simulink model "DAB_variableload"  (R2024b)
settings: Solver=VariableStepAuto  StartTime=0.0  StopTime=1  RelTol=1e-3
undefined symbols (not defined in the file): sigbuilder_block
libraries: spsMosfetLib x16, spsVoltageMeasurementLib x9, spsSeriesRLCBranchLib x7, spsCurrentMeasurementLib x6, simulink x5, slpidlib x4, spsMeanLib x4, spsParallelRLCBranchLib x4, spsRMSLib x4, spsDCVoltageSourceLib x2, spsLinearTransformerLib x2, spsControlledCurrentSourceLib x1
settings Model: Creator=shiekhsoliha  LastModifiedBy=sheikhsoliha
settings SolverCC: AlgebraicLoopSolver=TrustRegion
settings DataIOCC: ReturnWorkspaceOutputs=off
settings OptimizationCC: ReuseModelBlockBuffer=off  EfficientMapNaN2IntZero=off  AccelVerboseBuild=on
settings DebuggingCC: UnconnectedInputMsg=warning  UnconnectedOutputMsg=warning  UnconnectedLineMsg=warning  ArithmeticOperatorsInVariantConditions=warning
settings HardwareCC: TargetBitPerLong=64  TargetBitPerPointer=64  TargetBitPerSizeT=64  TargetBitPerPtrDiffT=64  TargetLongLongMode=on  TargetIntDivRoundTo=Zero  TargetEndianess=LittleEndian  TargetWordSize=64  TargetHWDeviceType=MATLAB Host  ProdEqTarget=off
settings ModelReferenceCC: EnableRefExpFcnMdlSchedulingChecks=on
settings SFSimCC: SimUseLocalCustomCode=off  CustomCodeUndefinedFunction=UseInterfaceOnly
settings RTWCC: RTWUseLocalCustomCode=off  GPUComputeCapability=3.5
settings CodeAppCC: MaxIdLength=128
settings GRTTargetCC: TargetLangStandard=C89/C90 (ANSI)  CombineOutputUpdateFcns=off  GRTInterface=on

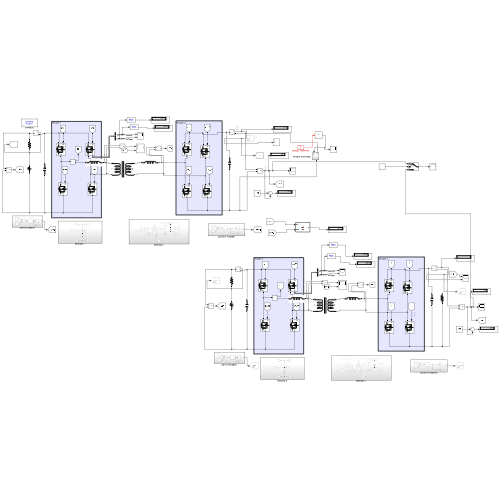
[thumbnail: Simulink's stored preview of the top-level diagram]
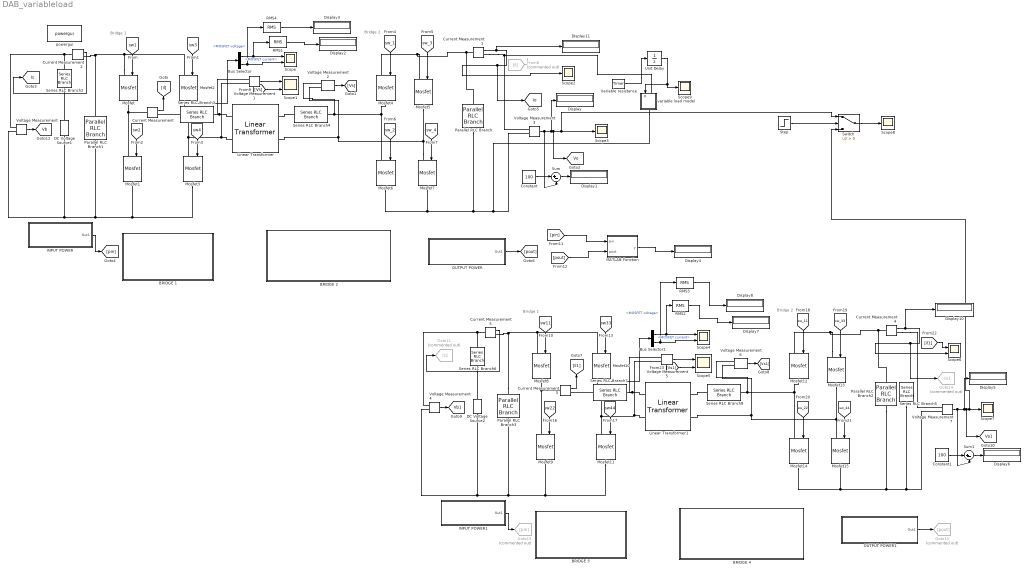
== system DAB_variableload ==
  note: Bridge 1
  note: Bridge 2
  note: Bridge 2
  note: Bridge 1
  " variable load model" : Subsystem
  BRIDGE 1 : Subsystem
  BRIDGE 2 : Subsystem
  BRIDGE 3 : Subsystem
  BRIDGE 4 : Subsystem
  Bus Selector : BusSelector  OutputSignals=MOSFET current,MOSFET voltage
  Bus Selector1 : BusSelector  OutputSignals=MOSFET current,MOSFET voltage
  Constant : Constant  Value=100
  Constant1 : Constant  Value=100
  Current Measurement{,1..5} (6 alike) : spsCurrentMeasurementLib/Current Measurement  PhasorSimulation=off  OutputType=Complex  PSBequivalent=0
  DC Voltage Source1 : spsDCVoltageSourceLib/DC Voltage Source  Amplitude=800  Measurements=None
  DC Voltage Source2 : spsDCVoltageSourceLib/DC Voltage Source  Amplitude=800  Measurements=None
  Display{,1..8,10..11} (11 alike) : Display
  From8 : From  Commented=on  GotoTag=il
  Goto11 : Goto  Commented=on  GotoTag=Is1  TagVisibility=global
  Goto13 : Goto  Commented=on  GotoTag=pin
  Goto14 : Goto  Commented=on  GotoTag=Io1  TagVisibility=global
  Goto15 : Goto  Commented=on  GotoTag=pout
  INPUT POWER : Subsystem
  INPUT POWER1 : Subsystem
  Linear Transformer : spsLinearTransformerLib/Linear Transformer  UNITS=pu  NominalPower=[ 2.5e3 50e3 ]  winding1=[1 0 0]  winding2=[1 0 0 ]  ThreeWindings=off  winding3=[ 315e3 0.002 0.08 ]  RmLm=[ 1e6 1e6 ]  Measurements=None  DataType=off
  Linear Transformer1 : spsLinearTransformerLib/Linear Transformer  UNITS=pu  NominalPower=[ 2.5e3 50e3 ]  winding1=[1 0 0]  winding2=[1 0 0 ]  ThreeWindings=off  winding3=[ 315e3 0.002 0.08 ]  RmLm=[ 1e6 1e6 ]  Measurements=None  DataType=off
  MATLAB Function : MATLAB Function  TreatAsAtomicUnit=on
  Mosfet{,1,3..9,11..15} (14 alike) : spsMosfetLib/Mosfet  Ron=0.1  Lon=0  Rd=0.01  Vfd=0  IC=0  Rs=1e5  Cs=inf  Measurements=off
  Mosfet10 : spsMosfetLib/Mosfet  Ron=0.1  Lon=0  Rd=0.01  Vfd=0  IC=0  Rs=1e5  Cs=inf  Measurements=on
  Mosfet2 : spsMosfetLib/Mosfet  Ron=0.1  Lon=0  Rd=0.01  Vfd=0  IC=0  Rs=1e5  Cs=inf  Measurements=on
  OUTPUT POWER : Subsystem
  OUTPUT POWER1 : Subsystem
  Parallel RLC Branch{,1..3} (4 alike) : spsParallelRLCBranchLib/Parallel RLC Branch  LConnTagsString=a  RConnTagsString=__new0  BranchType=C  Resistance=72.2  Inductance=1e-3  SetiL0=off  InitialCurrent=0  Capacitance=1.8e-3  Setx0=off  InitialVoltage=0  Measurements=None
  RMS{1..4} (4 alike) : spsRMSLib/RMS  TrueRMS=on  Freq=60  RMSInit=120  Ts=0
  Scope{,1,4..6} (5 alike) : Scope  NumInputPorts=2
  Scope{2..3,7..9} (5 alike) : Scope
  Series RLC Branch2 : spsSeriesRLCBranchLib/Series RLC Branch  LConnTagsString=__new0  RConnTagsString=__new0  BranchType=R  Resistance=0.1  Inductance=1e-3  SetiL0=off  InitialCurrent=0  Capacitance=1e-6  Setx0=off  InitialVoltage=0  Measurements=None
  Series RLC Branch{3..4,7..8} (4 alike) : spsSeriesRLCBranchLib/Series RLC Branch  LConnTagsString=__new0  RConnTagsString=__new0  BranchType=L  Resistance=0.1  Inductance=9.8e-6  SetiL0=off  InitialCurrent=0  Capacitance=1e-6  Setx0=off  InitialVoltage=0  Measurements=None
  Series RLC Branch5 : spsSeriesRLCBranchLib/Series RLC Branch  LConnTagsString=__new0  RConnTagsString=__new0  BranchType=R  Resistance=15  Inductance=1e-3  SetiL0=off  InitialCurrent=0  Capacitance=1e-6  Setx0=off  InitialVoltage=0  Measurements=None
  Series RLC Branch6 : spsSeriesRLCBranchLib/Series RLC Branch  LConnTagsString=__new0  RConnTagsString=__new0  BranchType=R  Resistance=0.1  Inductance=1e-3  SetiL0=off  InitialCurrent=0  Capacitance=1e-6  Setx0=off  InitialVoltage=0  Measurements=None
  Step : Step  Time=0.17  SampleTime=0
  Sum : Sum  Inputs=|+-
  Sum1 : Sum  Inputs=|+-
  Switch : Switch  Criteria=u2 > Threshold  SaturateOnIntegerOverflow=off  InputSameDT=off
  Unit Delay : UnitDelay  SampleTime=-1  HasFrameUpgradeWarning=on
  Variable resistance : powerlib_extras/Control  Blocks/Timer  t="[0  0.5 1]"  e=[31.2 15 15]
  Voltage Measurement{,1..7} (8 alike) : spsVoltageMeasurementLib/Voltage Measurement  PhasorSimulation=off  OutputType=Complex  PSBequivalent=0
  powergui : sps_lib/powergui  Priority=1  SimulationMode=Discrete  SampleTime=10e-7  frequency=60  Iterations=50  frequencyindice=0  Pbase=100e6  ErrMax=1e-4  UnitsV=kV  UnitsW=MW  buscounter=0  FunctionMessages=off  echomessages=off  EnableUseOfTLC=off  CurrentSourceSwitches=off  DisableSnubberDevices=off  DisableRonSwitches=off  DisableVfSwitches=off  DisplayEquations=off  AutomaticDiscreteSolvers=off  SolverType=Tustin/Backward Euler (TBE)  Interpol=off  ExternalGateDelay=off  methode=off  Ts=100  x0status=blocks  SPID=on  SwTol=0  HookPort=off  NonlinearTolerance=1e-4  nMaxIteration=100  ContinueOnMaxIteration=off  RestoreLinks=warning  ResistiveCurrentMeasurement=off  Frange=[0:2:500]  Ylog=off  Xlog=on  ShowGrid=off  save=off  variable=ZData  structure=0  ZoomFFT=off  StartTime=0.0  cycles=1  DisplayStyle=1  fundamental=60  FreqAxis=off  MaxFrequency=1000  frequencyindicesteady=1  RmsSteady=1  display=off
  tag scope: Io=global, Is=global, Vb1=global, Vb=global, Vo1=global, Vo=global
  wires:
  Voltage Measurement1/1 -> Scope1/1
  [sw_1] -> Mosfet4/1
  [sw_4] -> Mosfet7/1
  [sw_2] -> Mosfet6/1
  From8/1 -> ?
  [sw3] -> Mosfet2/1
  [sw_3] -> Mosfet5/1
  [Vs] -> Scope1/2
  Current Measurement/1 -> [il]
  [sw4] -> Mosfet3/1
  [sw1] -> Mosfet/1
  [sw2] -> Mosfet1/1
  Voltage Measurement2/1 -> [Vs]
  Voltage Measurement/1 -> [Vb]
  Constant/1 -> Sum/1
  Sum/1 -> Display1/1
  Mosfet2/1 -> Bus Selector/1
  Bus Selector/1 -> RMS1/1, Scope/1  "<MOSFET current>"
  Bus Selector/2 -> RMS4/1, Scope/2  "<MOSFET voltage>"
  RMS1/1 -> Display2/1
  RMS4/1 -> Display3/1
  Current Measurement2/1 -> [Is]
  INPUT POWER/1(Out1) -> [pin]
  OUTPUT POWER/1(Out1) -> [pout]
  [pin] -> MATLAB Function/1(pin)
  [pout] -> MATLAB Function/2(pout)
  MATLAB Function/1(y) -> Display4/1
  Voltage Measurement3/1 -> Sum/2, Display/1, [Vo], Switch/1, Scope3/1
  Step/1 -> Switch/2
  Voltage Measurement7/1 -> Sum1/2, Display5/1, [Vo1], Switch/3, Scope7/1
  [sw_11] -> Mosfet12/1
  [sw_22] -> Mosfet14/1
  Constant1/1 -> Sum1/1
  [sw11] -> Mosfet8/1
  [Vs1] -> Scope5/2
  Current Measurement3/1 -> [il1]
  Voltage Measurement5/1 -> Scope5/1
  Voltage Measurement4/1 -> [Vb1]
  [sw22] -> Mosfet9/1
  INPUT POWER1/1(Out1) -> Goto13/1
  Voltage Measurement6/1 -> [Vs1]
  Current Measurement5/1 -> Goto11/1
  OUTPUT POWER1/1(Out1) -> Goto15/1
  [il1] -> Scope6/1
  Current Measurement4/1 -> Display10/1, Goto14/1, Scope6/2
  [sw44] -> Mosfet11/1
  [sw_33] -> Mosfet13/1
  [sw_44] -> Mosfet15/1
  Mosfet10/1 -> Bus Selector1/1
  RMS2/1 -> Display7/1
  [sw33] -> Mosfet10/1
  Bus Selector1/2 -> RMS3/1, Scope4/2  "<MOSFET voltage>"
  RMS3/1 -> Display8/1
  Sum1/1 -> Display6/1
  Bus Selector1/1 -> RMS2/1, Scope4/1  "<MOSFET current>"
  Switch/1 -> Scope8/1
  Variable resistance/1 -> Unit Delay/1
  Unit Delay/1 -> Scope9/1, " variable load model"/1(R)
  Current Measurement1/1 -> Display11/1, [Io], Scope2/1
  connections:
  Mosfet/RConn1 -- Mosfet1/LConn1 -- Current Measurement/LConn1
  Mosfet2/RConn1 -- Voltage Measurement1/LConn2 -- Linear Transformer/LConn2 -- Mosfet3/LConn1
  Mosfet/LConn1 -- Mosfet2/LConn1 -- Current Measurement2/RConn1 -- Parallel RLC Branch1/LConn1
  Parallel RLC Branch1/RConn1 -- Voltage Measurement/LConn2 -- DC Voltage Source1/LConn1 -- Mosfet1/RConn1 -- Mosfet3/RConn1
  Current Measurement1/RConn1 -- " variable load model"/LConn1 -- Voltage Measurement3/LConn1
  Mosfet7/RConn1 -- Mosfet6/RConn1 -- Parallel RLC Branch/RConn1 -- " variable load model"/RConn1 -- Voltage Measurement3/LConn2
  Mosfet7/LConn1 -- Mosfet5/RConn1 -- Voltage Measurement2/LConn2 -- Linear Transformer/RConn2
  Voltage Measurement1/LConn1 -- Linear Transformer/LConn1 -- Series RLC Branch3/RConn1
  Series RLC Branch2/RConn1 -- DC Voltage Source1/RConn1
  Mosfet4/LConn1 -- Parallel RLC Branch/LConn1 -- Current Measurement1/LConn1 -- Mosfet5/LConn1
  Series RLC Branch3/LConn1 -- Current Measurement/RConn1
  Voltage Measurement2/LConn1 -- Mosfet6/LConn1 -- Mosfet4/RConn1 -- Series RLC Branch4/RConn1
  Series RLC Branch4/LConn1 -- Linear Transformer/RConn1
  Voltage Measurement/LConn1 -- Series RLC Branch2/LConn1 -- Current Measurement2/LConn1
  Mosfet11/LConn1 -- Mosfet10/RConn1 -- Voltage Measurement5/LConn2 -- Linear Transformer1/LConn2
  Mosfet13/LConn1 -- Mosfet12/LConn1 -- Parallel RLC Branch2/LConn1 -- Current Measurement4/LConn1
  Voltage Measurement6/LConn1 -- Series RLC Branch8/RConn1 -- Mosfet14/LConn1 -- Mosfet12/RConn1
  Voltage Measurement7/LConn2 -- Mosfet15/RConn1 -- Mosfet14/RConn1 -- Parallel RLC Branch2/RConn1 -- Series RLC Branch5/RConn1
  Linear Transformer1/RConn2 -- Mosfet15/LConn1 -- Mosfet13/RConn1 -- Voltage Measurement6/LConn2
  Current Measurement5/LConn1 -- Voltage Measurement4/LConn1 -- Series RLC Branch6/LConn1
  Current Measurement4/RConn1 -- Voltage Measurement7/LConn1
  DC Voltage Source2/LConn1 -- Parallel RLC Branch3/RConn1 -- Mosfet9/RConn1 -- Mosfet11/RConn1 -- Voltage Measurement4/LConn2
  Parallel RLC Branch3/LConn1 -- Current Measurement5/RConn1 -- Mosfet8/LConn1 -- Mosfet10/LConn1
  Series RLC Branch7/RConn1 -- Voltage Measurement5/LConn1 -- Linear Transformer1/LConn1
  Current Measurement3/LConn1 -- Mosfet8/RConn1 -- Mosfet9/LConn1
  Series RLC Branch6/RConn1 -- DC Voltage Source2/RConn1
  Series RLC Branch7/LConn1 -- Current Measurement3/RConn1
  Series RLC Branch8/LConn1 -- Linear Transformer1/RConn1

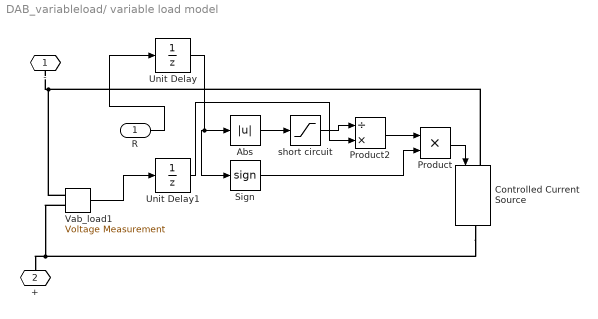
== system DAB_variableload/ variable load model ==
  R : Inport
  Abs : Abs  SampleTime=1e-06  SaturateOnIntegerOverflow=off
  Controlled Current Source : spsControlledCurrentSourceLib/Controlled Current Source  Initialize=on  Source_Type=AC  Amplitude=0  Phase=0  Frequency=0  Measurements=None
  Product : Product
  Product2 : Product  Inputs=/*  RndMeth=Zero
  Sign : Signum
  Unit Delay : UnitDelay  SampleTime=-1  HasFrameUpgradeWarning=on
  Unit Delay1 : UnitDelay  SampleTime=-1  HasFrameUpgradeWarning=on
  Vab_load1 : spsVoltageMeasurementLib/Voltage Measurement  Tag=PoWeRsYsTeMmEaSuReMeNt  PhasorSimulation=off  OutputType=Magnitude  PSBequivalent=0
  short circuit : Saturate  UpperLimit=164  LowerLimit=0.0001
  - : PMIOPort  Side=Right
  + : PMIOPort  Port=2  Side=Left
  wires:
  Product/1 -> Controlled Current Source/1
  short circuit/1 -> Product2/1
  Product2/1 -> Product/1
  Unit Delay/1 -> Sign/1, Abs/1
  Sign/1 -> Product/2
  Abs/1 -> short circuit/1
  Unit Delay1/1 -> Product2/2
  R/1 -> Unit Delay/1
  Vab_load1/1 -> Unit Delay1/1
  connections:
  Controlled Current Source/LConn1 -- Vab_load1/LConn1 -- -/RConn1
  Controlled Current Source/RConn1 -- +/RConn1 -- Vab_load1/LConn2

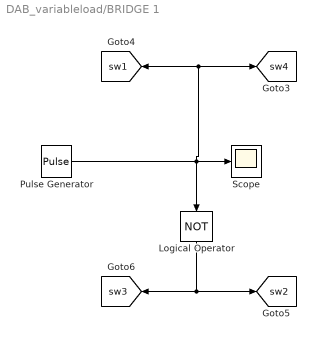
== system DAB_variableload/BRIDGE 1 ==
  Logical Operator : Logic  Operator=NOT  AllPortsSameDT=off  OutDataTypeStr=boolean
  Pulse Generator : DiscretePulseGenerator  PulseType=Time based  Period=1/50000  PulseWidth=50
  Scope : Scope
  tag scope: sw1=global, sw2=global, sw3=global, sw4=global
  wires:
  Logical Operator/1 -> [sw3], [sw2]
  Pulse Generator/1 -> Scope/1, [sw1], [sw4], Logical Operator/1

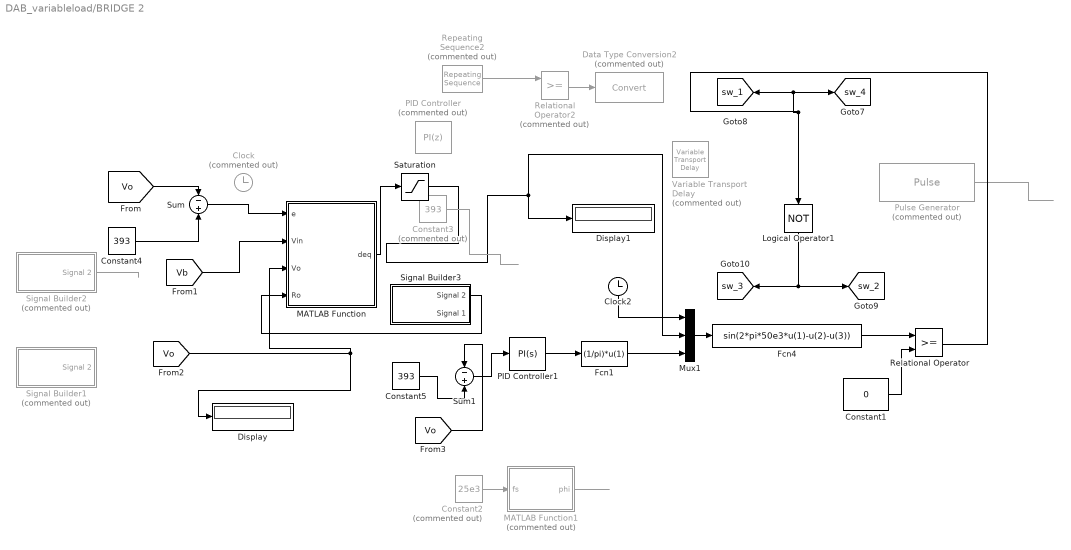
== system DAB_variableload/BRIDGE 2 ==
  Clock : Clock  Commented=on
  Clock2 : Clock
  Constant1 : Constant  Value=0
  Constant2 : Constant  Commented=on  Value=25e3
  Constant3 : Constant  Commented=on  Value=393
  Constant4 : Constant  Value=393
  Constant5 : Constant  Value=393
  Data Type Conversion2 : DataTypeConversion  Commented=on  SaturateOnIntegerOverflow=off  RndMeth=Floor
  Display : Display
  Display1 : Display
  Fcn1 : Fcn  Expr=(1/pi)*u(1)
  Fcn4 : Fcn  Expr=sin(2*pi*50e3*u(1)-u(2)-u(3))
  Logical Operator1 : Logic  Operator=NOT  AllPortsSameDT=off  OutDataTypeStr=boolean
  MATLAB Function : MATLAB Function  TreatAsAtomicUnit=on
  MATLAB Function1 : MATLAB Function  Commented=on  TreatAsAtomicUnit=on
  Mux1 : Mux  Inputs=3
  PID Controller : slpidlib/PID Controller  Commented=on  Controller=PI  Form=Parallel  TimeDomain=Discrete-time  UseExternalTs=off  SampleTime=-1  IntegratorMethod=Forward Euler  FilterMethod=Forward Euler  ControllerParametersSource=internal  P=0.0001  I=0.066  UseKiTs=off  D=0  UseExternalDerivativeSource=off  N=100  UseFilter=on  TunerSelectOption=Transfer Function Based (PID Tuner App)  InitialConditionSource=internal  InitialConditionForIntegrator=0  InitialConditionForFilter=0  DifferentiatorICPrevScaledInput=0  ExternalReset=none  TrackingMode=off  Kt=1  LimitOutput=on  SatLimitsSource=internal  UpperSaturationLimit=0.5  LowerSaturationLimit=0  LinearizeAsGain=on  AntiWindupMode=none  Kb=1  LimitIntegrator=off  UpperIntegratorSaturationLimit=inf  LowerIntegratorSaturationLimit=-inf  POutMin=[]  POutMax=[]  IOutMin=[]  IOutMax=[]  DOutMin=[]  DOutMax=[]  NOutMin=[]  NOutMax=[]  SumOutMin=[]  SumOutMax=[]  SaturationOutMin=[]  SaturationOutMax=[]  PParamMin=[]  PParamMax=[]  IParamMin=[]  IParamMax=[]  DParamMin=[]  DParamMax=[]  NParamMin=[]  NParamMax=[]  KbParamMin=[]  KbParamMax=[]  KtParamMin=[]  KtParamMax=[]  KbOutMin=[]  KbOutMax=[]  KtOutMin=[]  KtOutMax=[]  IntegratorOutMin=[]  IntegratorOutMax=[]  FilterOutMin=[]  FilterOutMax=[]  SumI1OutMin=[]  SumI1OutMax=[]  SumI2OutMin=[]  SumI2OutMax=[]  SumI3OutMin=[]  SumI3OutMax=[]  SumI4OutMin=[]  SumI4OutMax=[]  SumDOutMin=[]  SumDOutMax=[]  DifferentiatorOutMin=[]  DifferentiatorOutMax=[]  FilterDiffOutCoefMin=[]  FilterDiffOutCoefMax=[]  ReciprocalOutMin=[]  ReciprocalOutMax=[]  SumDenOutMin=[]  SumDenOutMax=[]  SumNumOutMin=[]  SumNumOutMax=[]  DivideOutMin=[]  DivideOutMax=[]  UdiffTsProdOutMin=[]  UdiffTsProdOutMax=[]  NTsProdOutMin=[]  NTsProdOutMax=[]  UintegralTsProdOutMin=[]  UintegralTsProdOutMax=[]  UngainTsProdOutMin=[]  UngainTsProdOutMax=[]  ClampingZeroOutDataTypeStr=Inherit: Inherit via back propagation  ClampingZeroOutMin=[]  ClampingZeroOutMax=[]  FilterDenConstantOutDataTypeStr=Inherit: Inherit via back propagation  FilterDenConstantOutMin=[]  FilterDenConstantOutMax=[]  PCopyOutDataTypeStr=Inherit: Inherit via back propagation  PCopyOutMin=[]  PCopyOutMax=[]  NCopyOutDataTypeStr=Inherit: Inherit via back propagation  NCopyOutMin=[]  NCopyOutMax=[]  IntegratorContinuousStateAttributes=''  IntegratorStateMustResolveToSignalObject=off  IntegratorRTWStateStorageClass=Auto  FilterContinuousStateAttributes=''  FilterStateMustResolveToSignalObject=off  FilterRTWStateStorageClass=Auto  ParallelPVariant=InternalParameters  IdealPVariant=Disabled  IVariant=InternalParameters  DVariant=Disabled  IntegratorVariant=Discrete  SatVariant=Enabled  AWVariant=Passthrough  PCopyVariant=Disabled  TRVariant=Disabled  FdbkBlocksVariant=Forward  IdealPFdbkVariant=Disabled  SatFdbkVariant=Disabled  DerivativeFilterVariant=Disabled  NVariant=Disabled  NCopyVariant=Disabled_SignalSpec  FilterICVariant=Disabled  IntegratorICVariant=InternalICs  ExternalResetVariant=Disabled  TRSumVariant=Passthrough  SumFdbkVariant=Disabled  SumVariant=Sum_PI  TsampFilterVariant=InternalTs  TsampNgainVariant=Passthrough  TsampIntegralVariant=Disabled_SignalSpec  ExternalSaturationOutDataTypeStr=Inherit: Same as second input  DerivativeSourceVariant=Disabled  PreIntVariant=InternalPreInt
  PID Controller1 : slpidlib/PID Controller  Controller=PI  Form=Parallel  TimeDomain=Continuous-time  UseExternalTs=off  SampleTime=-1  IntegratorMethod=Forward Euler  FilterMethod=Forward Euler  ControllerParametersSource=internal  P=0.037  I=4.65  UseKiTs=off  D=0  UseExternalDerivativeSource=off  N=100  UseFilter=on  TunerSelectOption=Transfer Function Based (PID Tuner App)  InitialConditionSource=internal  InitialConditionForIntegrator=0  InitialConditionForFilter=0  DifferentiatorICPrevScaledInput=0  ExternalReset=none  TrackingMode=off  Kt=1  LimitOutput=on  SatLimitsSource=internal  UpperSaturationLimit=393  LowerSaturationLimit=0  LinearizeAsGain=on  AntiWindupMode=none  Kb=1  LimitIntegrator=off  UpperIntegratorSaturationLimit=inf  LowerIntegratorSaturationLimit=-inf  POutMin=[]  POutMax=[]  IOutMin=[]  IOutMax=[]  DOutMin=[]  DOutMax=[]  NOutMin=[]  NOutMax=[]  SumOutMin=[]  SumOutMax=[]  SaturationOutMin=[]  SaturationOutMax=[]  PParamMin=[]  PParamMax=[]  IParamMin=[]  IParamMax=[]  DParamMin=[]  DParamMax=[]  NParamMin=[]  NParamMax=[]  KbParamMin=[]  KbParamMax=[]  KtParamMin=[]  KtParamMax=[]  KbOutMin=[]  KbOutMax=[]  KtOutMin=[]  KtOutMax=[]  IntegratorOutMin=[]  IntegratorOutMax=[]  FilterOutMin=[]  FilterOutMax=[]  SumI1OutMin=[]  SumI1OutMax=[]  SumI2OutMin=[]  SumI2OutMax=[]  SumI3OutMin=[]  SumI3OutMax=[]  SumI4OutMin=[]  SumI4OutMax=[]  SumDOutMin=[]  SumDOutMax=[]  DifferentiatorOutMin=[]  DifferentiatorOutMax=[]  FilterDiffOutCoefMin=[]  FilterDiffOutCoefMax=[]  ReciprocalOutMin=[]  ReciprocalOutMax=[]  SumDenOutMin=[]  SumDenOutMax=[]  SumNumOutMin=[]  SumNumOutMax=[]  DivideOutMin=[]  DivideOutMax=[]  UdiffTsProdOutMin=[]  UdiffTsProdOutMax=[]  NTsProdOutMin=[]  NTsProdOutMax=[]  UintegralTsProdOutMin=[]  UintegralTsProdOutMax=[]  UngainTsProdOutMin=[]  UngainTsProdOutMax=[]  ClampingZeroOutDataTypeStr=Inherit: Inherit via back propagation  ClampingZeroOutMin=[]  ClampingZeroOutMax=[]  FilterDenConstantOutDataTypeStr=Inherit: Inherit via back propagation  FilterDenConstantOutMin=[]  FilterDenConstantOutMax=[]  PCopyOutDataTypeStr=Inherit: Inherit via back propagation  PCopyOutMin=[]  PCopyOutMax=[]  NCopyOutDataTypeStr=Inherit: Inherit via back propagation  NCopyOutMin=[]  NCopyOutMax=[]  IntegratorContinuousStateAttributes=''  IntegratorStateMustResolveToSignalObject=off  IntegratorRTWStateStorageClass=Auto  FilterContinuousStateAttributes=''  FilterStateMustResolveToSignalObject=off  FilterRTWStateStorageClass=Auto  ParallelPVariant=InternalParameters  IdealPVariant=Disabled  IVariant=InternalParameters  DVariant=Disabled  IntegratorVariant=Continuous  SatVariant=Enabled  AWVariant=Passthrough  PCopyVariant=Disabled  TRVariant=Disabled  FdbkBlocksVariant=Forward  IdealPFdbkVariant=Disabled  SatFdbkVariant=Disabled  DerivativeFilterVariant=Disabled  NVariant=Disabled  NCopyVariant=Disabled_SignalSpec  FilterICVariant=Disabled  IntegratorICVariant=InternalICs  ExternalResetVariant=Disabled  TRSumVariant=Passthrough  SumFdbkVariant=Disabled  SumVariant=Sum_PI  TsampFilterVariant=InternalTs  TsampNgainVariant=Passthrough  TsampIntegralVariant=Disabled_SignalSpec  ExternalSaturationOutDataTypeStr=Inherit: Same as second input  DerivativeSourceVariant=Disabled  PreIntVariant=InternalPreInt
  Pulse Generator : DiscretePulseGenerator  Commented=on  PulseType=Time based  Period=1/50000  PulseWidth=50
  Relational Operator : RelationalOperator  OutDataTypeStr=boolean  RndMeth=Simplest  InputSameDT=off
  Relational Operator2 : RelationalOperator  Commented=on  OutDataTypeStr=boolean  InputSameDT=off
  Repeating Sequence2 : simulink/Sources/Repeating Sequence  Commented=on  rep_seq_t=[0 1/50000]  rep_seq_y=[0 1]
  Saturation : Saturate  LowerLimit=0
  Signal Builder1 : Subsystem  Tag=STV Subsys  Commented=on  LoadFcn=sigbuilder_block('load');  StartFcn=sigbuilder_block('start');  StopFcn=sigbuilder_block('stop');  ClipboardFcn=sigbuilder_block('clipboard');  mask(Sigbuilder block){tuvar=[0:10]}
      mask help: Simulink:masks:SigbuilderBlock_MD
      mask init:
      | if ~strcmp(get_param(bdroot(gcbh),'SimulationStatus'),'stopped') tuvar = sigbuilder_block('maskInit'); end
      settings: CopyFcn=sigbuilder_block('copy');  DeleteFcn=sigbuilder_block('delete');  ModelCloseFcn=sigbuilder_block('modelClose');  PreSaveFcn=sigbuilder_block('preSave');  PauseFcn=sigbuilder_block('pause');  ContinueFcn=sigbuilder_block('continue');  NameChangeFcn=sigbuilder_block('namechange');  OpenFcn=sigbuilder_block('open',[437.6 199.2 550.4 400 ]);  CloseFcn=sigbuilder_block('close');
      mask Display: plot(0, 0, 100, 100,[2, 2, 32, 32, 2], [68, 8, 8, 68, 68],[32, 2], [38, 38], [32, 19, 2],[53, 60, 44], [32, 17, 17, 2],[16, 16, 31, 31]);txt = getActiveGroup(gcbh);text(2, 100, txt,'verticalAlignment', 'top');
  Signal Builder2 : Subsystem  Tag=STV Subsys  Commented=on  LoadFcn=sigbuilder_block('load');  StartFcn=sigbuilder_block('start');  StopFcn=sigbuilder_block('stop');  ClipboardFcn=sigbuilder_block('clipboard');  mask(Sigbuilder block){tuvar=[0:10]}
      mask help: Simulink:masks:SigbuilderBlock_MD
      mask init:
      | if ~strcmp(get_param(bdroot(gcbh),'SimulationStatus'),'stopped') tuvar = sigbuilder_block('maskInit'); end
      settings: CopyFcn=sigbuilder_block('copy');  DeleteFcn=sigbuilder_block('delete');  ModelCloseFcn=sigbuilder_block('modelClose');  PreSaveFcn=sigbuilder_block('preSave');  PauseFcn=sigbuilder_block('pause');  ContinueFcn=sigbuilder_block('continue');  NameChangeFcn=sigbuilder_block('namechange');  OpenFcn=sigbuilder_block('open',[437.6 199.2 550.4 400 ]);  CloseFcn=sigbuilder_block('close');
      mask Display: plot(0, 0, 100, 100,[2, 2, 32, 32, 2], [68, 8, 8, 68, 68],[32, 2], [38, 38], [32, 19, 2],[53, 60, 44], [32, 17, 17, 2],[16, 16, 31, 31]);txt = getActiveGroup(gcbh);text(2, 100, txt,'verticalAlignment', 'top');
  Signal Builder3 : Subsystem  Tag=STV Subsys  LoadFcn=sigbuilder_block('load');  StartFcn=sigbuilder_block('start');  StopFcn=sigbuilder_block('stop');  ClipboardFcn=sigbuilder_block('clipboard');  mask(Sigbuilder block){tuvar=[0:10]}
      mask help: Simulink:masks:SigbuilderBlock_MD
      mask init:
      | if ~strcmp(get_param(bdroot(gcbh),'SimulationStatus'),'stopped') tuvar = sigbuilder_block('maskInit'); end
      settings: CopyFcn=sigbuilder_block('copy');  DeleteFcn=sigbuilder_block('delete');  ModelCloseFcn=sigbuilder_block('modelClose');  PreSaveFcn=sigbuilder_block('preSave');  PauseFcn=sigbuilder_block('pause');  ContinueFcn=sigbuilder_block('continue');  NameChangeFcn=sigbuilder_block('namechange');  OpenFcn=sigbuilder_block('open',[0 62 1440 734 ]);  CloseFcn=sigbuilder_block('close');
      mask Display: plot(0, 0, 100, 100,[2, 2, 32, 32, 2], [68, 8, 8, 68, 68],[32, 2], [38, 38], [32, 19, 2],[53, 60, 44], [32, 17, 17, 2],[16, 16, 31, 31]);txt = getActiveGroup(gcbh);text(2, 100, txt,'verticalAlignment', 'top');
  Sum : Sum  Inputs=-+
  Sum1 : Sum  Inputs=-+
  Variable Transport Delay : VariableTransportDelay  Commented=on  VariableDelayType=Variable transport delay  MaximumDelay=3e-3
  tag scope: sw_1=global, sw_2=global, sw_3=global, sw_4=global
  wires:
  Sum/1 -> MATLAB Function/1(e)
  [Vb] -> MATLAB Function/2(Vin)
  Logical Operator1/1 -> [sw_2], [sw_3]
  [Vo] -> MATLAB Function/3(Vo), Display/1
  Relational Operator2/1 -> Data Type Conversion2/1
  Repeating Sequence2/1 -> Relational Operator2/1
  Constant2/1 -> MATLAB Function1/1(fs)
  Fcn4/1 -> Relational Operator/1
  Constant1/1 -> Relational Operator/2
  Mux1/1 -> Fcn4/1
  MATLAB Function1/1(phi) -> ?
  Clock2/1 -> Mux1/1
  [Vo] -> Sum1/1
  Sum1/1 -> PID Controller1/1
  Pulse Generator/1 -> ?
  Saturation/1 -> Mux1/2, Display1/1
  Relational Operator/1 -> [sw_1], [sw_4], Logical Operator1/1
  Constant3/1 -> ?
  PID Controller1/1 -> Fcn1/1
  Fcn1/1 -> Mux1/3
  [Vo] -> Sum/1
  Signal Builder2/1(Signal 2) -> ?
  Constant4/1 -> Sum/2
  Signal Builder3/1(Signal 2) -> MATLAB Function/4(Ro)
  Constant5/1 -> Sum1/2
  MATLAB Function/1(deq) -> Saturation/1

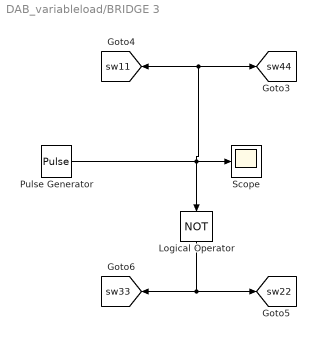
== system DAB_variableload/BRIDGE 3 ==
  Logical Operator : Logic  Operator=NOT  AllPortsSameDT=off  OutDataTypeStr=boolean
  Pulse Generator : DiscretePulseGenerator  PulseType=Time based  Period=1/50000  PulseWidth=50
  Scope : Scope
  tag scope: sw11=global, sw22=global, sw33=global, sw44=global
  wires:
  Logical Operator/1 -> [sw33], [sw22]
  Pulse Generator/1 -> Scope/1, [sw11], [sw44], Logical Operator/1

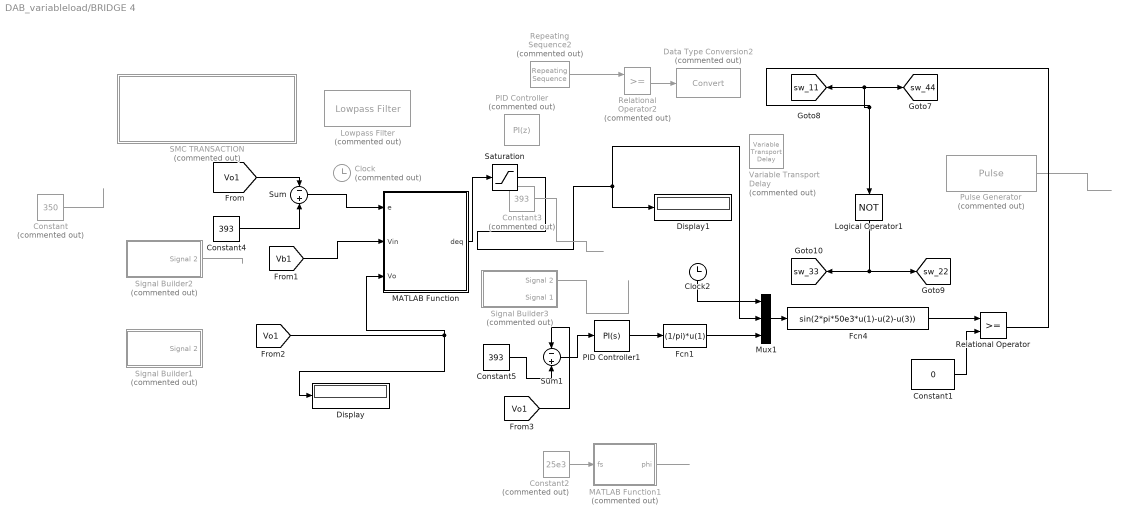
== system DAB_variableload/BRIDGE 4 ==
  Clock : Clock  Commented=on
  Clock2 : Clock
  Constant : Constant  Commented=on  Value=350
  Constant1 : Constant  Value=0
  Constant2 : Constant  Commented=on  Value=25e3
  Constant3 : Constant  Commented=on  Value=393
  Constant4 : Constant  Value=393
  Constant5 : Constant  Value=393
  Data Type Conversion2 : DataTypeConversion  Commented=on  SaturateOnIntegerOverflow=off  RndMeth=Floor
  Display : Display
  Display1 : Display
  Fcn1 : Fcn  Expr=(1/pi)*u(1)
  Fcn4 : Fcn  Expr=sin(2*pi*50e3*u(1)-u(2)-u(3))
  Logical Operator1 : Logic  Operator=NOT  AllPortsSameDT=off  OutDataTypeStr=boolean
  Lowpass Filter : dspfdesign/Lowpass Filter  Commented=on  FilterType=FIR  DesignForMinimumOrder=on  FilterOrder=50  PassbandFrequency=8e3  StopbandFrequency=12e3  PassbandRipple=0.1  StopbandAttenuation=80  InheritSampleRate=off  SampleRate=44100  SimulateUsing=Interpreted execution  roundingMode=Floor  coeffsDataTypeStr=fixdt(1,16)
  MATLAB Function : MATLAB Function  TreatAsAtomicUnit=on
  MATLAB Function1 : MATLAB Function  Commented=on  TreatAsAtomicUnit=on
  Mux1 : Mux  Inputs=3
  PID Controller : slpidlib/PID Controller  Commented=on  Controller=PI  Form=Parallel  TimeDomain=Discrete-time  UseExternalTs=off  SampleTime=-1  IntegratorMethod=Forward Euler  FilterMethod=Forward Euler  ControllerParametersSource=internal  P=0.0001  I=0.066  UseKiTs=off  D=0  UseExternalDerivativeSource=off  N=100  UseFilter=on  TunerSelectOption=Transfer Function Based (PID Tuner App)  InitialConditionSource=internal  InitialConditionForIntegrator=0  InitialConditionForFilter=0  DifferentiatorICPrevScaledInput=0  ExternalReset=none  TrackingMode=off  Kt=1  LimitOutput=on  SatLimitsSource=internal  UpperSaturationLimit=0.5  LowerSaturationLimit=0  LinearizeAsGain=on  AntiWindupMode=none  Kb=1  LimitIntegrator=off  UpperIntegratorSaturationLimit=inf  LowerIntegratorSaturationLimit=-inf  POutMin=[]  POutMax=[]  IOutMin=[]  IOutMax=[]  DOutMin=[]  DOutMax=[]  NOutMin=[]  NOutMax=[]  SumOutMin=[]  SumOutMax=[]  SaturationOutMin=[]  SaturationOutMax=[]  PParamMin=[]  PParamMax=[]  IParamMin=[]  IParamMax=[]  DParamMin=[]  DParamMax=[]  NParamMin=[]  NParamMax=[]  KbParamMin=[]  KbParamMax=[]  KtParamMin=[]  KtParamMax=[]  KbOutMin=[]  KbOutMax=[]  KtOutMin=[]  KtOutMax=[]  IntegratorOutMin=[]  IntegratorOutMax=[]  FilterOutMin=[]  FilterOutMax=[]  SumI1OutMin=[]  SumI1OutMax=[]  SumI2OutMin=[]  SumI2OutMax=[]  SumI3OutMin=[]  SumI3OutMax=[]  SumI4OutMin=[]  SumI4OutMax=[]  SumDOutMin=[]  SumDOutMax=[]  DifferentiatorOutMin=[]  DifferentiatorOutMax=[]  FilterDiffOutCoefMin=[]  FilterDiffOutCoefMax=[]  ReciprocalOutMin=[]  ReciprocalOutMax=[]  SumDenOutMin=[]  SumDenOutMax=[]  SumNumOutMin=[]  SumNumOutMax=[]  DivideOutMin=[]  DivideOutMax=[]  UdiffTsProdOutMin=[]  UdiffTsProdOutMax=[]  NTsProdOutMin=[]  NTsProdOutMax=[]  UintegralTsProdOutMin=[]  UintegralTsProdOutMax=[]  UngainTsProdOutMin=[]  UngainTsProdOutMax=[]  ClampingZeroOutDataTypeStr=Inherit: Inherit via back propagation  ClampingZeroOutMin=[]  ClampingZeroOutMax=[]  FilterDenConstantOutDataTypeStr=Inherit: Inherit via back propagation  FilterDenConstantOutMin=[]  FilterDenConstantOutMax=[]  PCopyOutDataTypeStr=Inherit: Inherit via back propagation  PCopyOutMin=[]  PCopyOutMax=[]  NCopyOutDataTypeStr=Inherit: Inherit via back propagation  NCopyOutMin=[]  NCopyOutMax=[]  IntegratorContinuousStateAttributes=''  IntegratorStateMustResolveToSignalObject=off  IntegratorRTWStateStorageClass=Auto  FilterContinuousStateAttributes=''  FilterStateMustResolveToSignalObject=off  FilterRTWStateStorageClass=Auto  ParallelPVariant=InternalParameters  IdealPVariant=Disabled  IVariant=InternalParameters  DVariant=Disabled  IntegratorVariant=Discrete  SatVariant=Enabled  AWVariant=Passthrough  PCopyVariant=Disabled  TRVariant=Disabled  FdbkBlocksVariant=Forward  IdealPFdbkVariant=Disabled  SatFdbkVariant=Disabled  DerivativeFilterVariant=Disabled  NVariant=Disabled  NCopyVariant=Disabled_SignalSpec  FilterICVariant=Disabled  IntegratorICVariant=InternalICs  ExternalResetVariant=Disabled  TRSumVariant=Passthrough  SumFdbkVariant=Disabled  SumVariant=Sum_PI  TsampFilterVariant=InternalTs  TsampNgainVariant=Passthrough  TsampIntegralVariant=Disabled_SignalSpec  ExternalSaturationOutDataTypeStr=Inherit: Same as second input  DerivativeSourceVariant=Disabled  PreIntVariant=InternalPreInt
  PID Controller1 : slpidlib/PID Controller  Controller=PI  Form=Parallel  TimeDomain=Continuous-time  UseExternalTs=off  SampleTime=-1  IntegratorMethod=Forward Euler  FilterMethod=Forward Euler  ControllerParametersSource=internal  P=0.037  I=4.65  UseKiTs=off  D=0  UseExternalDerivativeSource=off  N=100  UseFilter=on  TunerSelectOption=Transfer Function Based (PID Tuner App)  InitialConditionSource=internal  InitialConditionForIntegrator=0  InitialConditionForFilter=0  DifferentiatorICPrevScaledInput=0  ExternalReset=none  TrackingMode=off  Kt=1  LimitOutput=on  SatLimitsSource=internal  UpperSaturationLimit=393  LowerSaturationLimit=0  LinearizeAsGain=on  AntiWindupMode=none  Kb=1  LimitIntegrator=off  UpperIntegratorSaturationLimit=inf  LowerIntegratorSaturationLimit=-inf  POutMin=[]  POutMax=[]  IOutMin=[]  IOutMax=[]  DOutMin=[]  DOutMax=[]  NOutMin=[]  NOutMax=[]  SumOutMin=[]  SumOutMax=[]  SaturationOutMin=[]  SaturationOutMax=[]  PParamMin=[]  PParamMax=[]  IParamMin=[]  IParamMax=[]  DParamMin=[]  DParamMax=[]  NParamMin=[]  NParamMax=[]  KbParamMin=[]  KbParamMax=[]  KtParamMin=[]  KtParamMax=[]  KbOutMin=[]  KbOutMax=[]  KtOutMin=[]  KtOutMax=[]  IntegratorOutMin=[]  IntegratorOutMax=[]  FilterOutMin=[]  FilterOutMax=[]  SumI1OutMin=[]  SumI1OutMax=[]  SumI2OutMin=[]  SumI2OutMax=[]  SumI3OutMin=[]  SumI3OutMax=[]  SumI4OutMin=[]  SumI4OutMax=[]  SumDOutMin=[]  SumDOutMax=[]  DifferentiatorOutMin=[]  DifferentiatorOutMax=[]  FilterDiffOutCoefMin=[]  FilterDiffOutCoefMax=[]  ReciprocalOutMin=[]  ReciprocalOutMax=[]  SumDenOutMin=[]  SumDenOutMax=[]  SumNumOutMin=[]  SumNumOutMax=[]  DivideOutMin=[]  DivideOutMax=[]  UdiffTsProdOutMin=[]  UdiffTsProdOutMax=[]  NTsProdOutMin=[]  NTsProdOutMax=[]  UintegralTsProdOutMin=[]  UintegralTsProdOutMax=[]  UngainTsProdOutMin=[]  UngainTsProdOutMax=[]  ClampingZeroOutDataTypeStr=Inherit: Inherit via back propagation  ClampingZeroOutMin=[]  ClampingZeroOutMax=[]  FilterDenConstantOutDataTypeStr=Inherit: Inherit via back propagation  FilterDenConstantOutMin=[]  FilterDenConstantOutMax=[]  PCopyOutDataTypeStr=Inherit: Inherit via back propagation  PCopyOutMin=[]  PCopyOutMax=[]  NCopyOutDataTypeStr=Inherit: Inherit via back propagation  NCopyOutMin=[]  NCopyOutMax=[]  IntegratorContinuousStateAttributes=''  IntegratorStateMustResolveToSignalObject=off  IntegratorRTWStateStorageClass=Auto  FilterContinuousStateAttributes=''  FilterStateMustResolveToSignalObject=off  FilterRTWStateStorageClass=Auto  ParallelPVariant=InternalParameters  IdealPVariant=Disabled  IVariant=InternalParameters  DVariant=Disabled  IntegratorVariant=Continuous  SatVariant=Enabled  AWVariant=Passthrough  PCopyVariant=Disabled  TRVariant=Disabled  FdbkBlocksVariant=Forward  IdealPFdbkVariant=Disabled  SatFdbkVariant=Disabled  DerivativeFilterVariant=Disabled  NVariant=Disabled  NCopyVariant=Disabled_SignalSpec  FilterICVariant=Disabled  IntegratorICVariant=InternalICs  ExternalResetVariant=Disabled  TRSumVariant=Passthrough  SumFdbkVariant=Disabled  SumVariant=Sum_PI  TsampFilterVariant=InternalTs  TsampNgainVariant=Passthrough  TsampIntegralVariant=Disabled_SignalSpec  ExternalSaturationOutDataTypeStr=Inherit: Same as second input  DerivativeSourceVariant=Disabled  PreIntVariant=InternalPreInt
  Pulse Generator : DiscretePulseGenerator  Commented=on  PulseType=Time based  Period=1/50000  PulseWidth=50
  Relational Operator : RelationalOperator  OutDataTypeStr=boolean  RndMeth=Simplest  InputSameDT=off
  Relational Operator2 : RelationalOperator  Commented=on  OutDataTypeStr=boolean  InputSameDT=off
  Repeating Sequence2 : simulink/Sources/Repeating Sequence  Commented=on  rep_seq_t=[0 1/50000]  rep_seq_y=[0 1]
  SMC TRANSACTION : Subsystem  Commented=on
  Saturation : Saturate  LowerLimit=0
  Signal Builder1 : Subsystem  Tag=STV Subsys  Commented=on  LoadFcn=sigbuilder_block('load');  StartFcn=sigbuilder_block('start');  StopFcn=sigbuilder_block('stop');  ClipboardFcn=sigbuilder_block('clipboard');  mask(Sigbuilder block){tuvar=[0:10]}
      mask help: Simulink:masks:SigbuilderBlock_MD
      mask init:
      | if ~strcmp(get_param(bdroot(gcbh),'SimulationStatus'),'stopped') tuvar = sigbuilder_block('maskInit'); end
      settings: CopyFcn=sigbuilder_block('copy');  DeleteFcn=sigbuilder_block('delete');  ModelCloseFcn=sigbuilder_block('modelClose');  PreSaveFcn=sigbuilder_block('preSave');  PauseFcn=sigbuilder_block('pause');  ContinueFcn=sigbuilder_block('continue');  NameChangeFcn=sigbuilder_block('namechange');  OpenFcn=sigbuilder_block('open',[437.6 199.2 550.4 400 ]);  CloseFcn=sigbuilder_block('close');
      mask Display: plot(0, 0, 100, 100,[2, 2, 32, 32, 2], [68, 8, 8, 68, 68],[32, 2], [38, 38], [32, 19, 2],[53, 60, 44], [32, 17, 17, 2],[16, 16, 31, 31]);txt = getActiveGroup(gcbh);text(2, 100, txt,'verticalAlignment', 'top');
  Signal Builder2 : Subsystem  Tag=STV Subsys  Commented=on  LoadFcn=sigbuilder_block('load');  StartFcn=sigbuilder_block('start');  StopFcn=sigbuilder_block('stop');  ClipboardFcn=sigbuilder_block('clipboard');  mask(Sigbuilder block){tuvar=[0:10]}
      mask help: Simulink:masks:SigbuilderBlock_MD
      mask init:
      | if ~strcmp(get_param(bdroot(gcbh),'SimulationStatus'),'stopped') tuvar = sigbuilder_block('maskInit'); end
      settings: CopyFcn=sigbuilder_block('copy');  DeleteFcn=sigbuilder_block('delete');  ModelCloseFcn=sigbuilder_block('modelClose');  PreSaveFcn=sigbuilder_block('preSave');  PauseFcn=sigbuilder_block('pause');  ContinueFcn=sigbuilder_block('continue');  NameChangeFcn=sigbuilder_block('namechange');  OpenFcn=sigbuilder_block('open',[437.6 199.2 550.4 400 ]);  CloseFcn=sigbuilder_block('close');
      mask Display: plot(0, 0, 100, 100,[2, 2, 32, 32, 2], [68, 8, 8, 68, 68],[32, 2], [38, 38], [32, 19, 2],[53, 60, 44], [32, 17, 17, 2],[16, 16, 31, 31]);txt = getActiveGroup(gcbh);text(2, 100, txt,'verticalAlignment', 'top');
  Signal Builder3 : Subsystem  Tag=STV Subsys  Commented=on  LoadFcn=sigbuilder_block('load');  StartFcn=sigbuilder_block('start');  StopFcn=sigbuilder_block('stop');  ClipboardFcn=sigbuilder_block('clipboard');  mask(Sigbuilder block){tuvar=[0:10]}
      mask help: Simulink:masks:SigbuilderBlock_MD
      mask init:
      | if ~strcmp(get_param(bdroot(gcbh),'SimulationStatus'),'stopped') tuvar = sigbuilder_block('maskInit'); end
      settings: CopyFcn=sigbuilder_block('copy');  DeleteFcn=sigbuilder_block('delete');  ModelCloseFcn=sigbuilder_block('modelClose');  PreSaveFcn=sigbuilder_block('preSave');  PauseFcn=sigbuilder_block('pause');  ContinueFcn=sigbuilder_block('continue');  NameChangeFcn=sigbuilder_block('namechange');  OpenFcn=sigbuilder_block('open',[0 71 1440 725 ]);  CloseFcn=sigbuilder_block('close');
      mask Display: plot(0, 0, 100, 100,[2, 2, 32, 32, 2], [68, 8, 8, 68, 68],[32, 2], [38, 38], [32, 19, 2],[53, 60, 44], [32, 17, 17, 2],[16, 16, 31, 31]);txt = getActiveGroup(gcbh);text(2, 100, txt,'verticalAlignment', 'top');
  Sum : Sum  Inputs=-+
  Sum1 : Sum  Inputs=-+
  Variable Transport Delay : VariableTransportDelay  Commented=on  VariableDelayType=Variable transport delay  MaximumDelay=3e-3
  tag scope: sw_11=global, sw_22=global, sw_33=global, sw_44=global
  wires:
  Constant/1 -> ?
  Sum/1 -> MATLAB Function/1(e)
  [Vb1] -> MATLAB Function/2(Vin)
  Logical Operator1/1 -> [sw_22], [sw_33]
  [Vo1] -> MATLAB Function/3(Vo), Display/1
  Relational Operator2/1 -> Data Type Conversion2/1
  Repeating Sequence2/1 -> Relational Operator2/1
  Constant2/1 -> MATLAB Function1/1(fs)
  Fcn4/1 -> Relational Operator/1
  Constant1/1 -> Relational Operator/2
  Mux1/1 -> Fcn4/1
  MATLAB Function1/1(phi) -> ?
  Clock2/1 -> Mux1/1
  [Vo1] -> Sum1/1
  Sum1/1 -> PID Controller1/1
  Pulse Generator/1 -> ?
  Saturation/1 -> Mux1/2, Display1/1
  Relational Operator/1 -> [sw_11], [sw_44], Logical Operator1/1
  Constant3/1 -> ?
  PID Controller1/1 -> Fcn1/1
  Fcn1/1 -> Mux1/3
  [Vo1] -> Sum/1
  Signal Builder2/1(Signal 2) -> ?
  Constant4/1 -> Sum/2
  Signal Builder3/1(Signal 2) -> ?
  Constant5/1 -> Sum1/2
  MATLAB Function/1(deq) -> Saturation/1

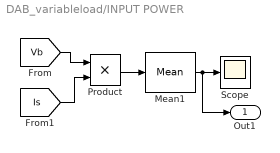
== system DAB_variableload/INPUT POWER ==
  Mean1 : spsMeanLib/Mean  Freq=60  Vinit=0  Ts=0
  Product : Product
  Scope : Scope
  Out1 : Outport  VectorParamsAs1DForOutWhenUnconnected=off
  wires:
  [Is] -> Product/2
  [Vb] -> Product/1
  Product/1 -> Mean1/1
  Mean1/1 -> Out1/1, Scope/1

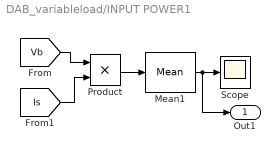
== system DAB_variableload/INPUT POWER1 ==
  Mean1 : spsMeanLib/Mean  Freq=60  Vinit=0  Ts=0
  Product : Product
  Scope : Scope
  Out1 : Outport  VectorParamsAs1DForOutWhenUnconnected=off
  wires:
  [Is] -> Product/2
  [Vb] -> Product/1
  Product/1 -> Mean1/1
  Mean1/1 -> Out1/1, Scope/1

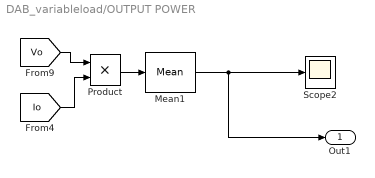
== system DAB_variableload/OUTPUT POWER ==
  Mean1 : spsMeanLib/Mean  Freq=60  Vinit=0  Ts=0
  Product : Product
  Scope2 : Scope
  Out1 : Outport  VectorParamsAs1DForOutWhenUnconnected=off
  wires:
  [Io] -> Product/2
  Mean1/1 -> Out1/1, Scope2/1
  Product/1 -> Mean1/1
  [Vo] -> Product/1

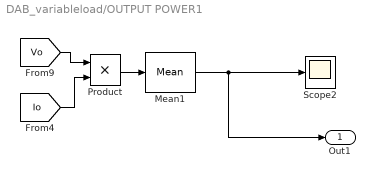
== system DAB_variableload/OUTPUT POWER1 ==
  Mean1 : spsMeanLib/Mean  Freq=60  Vinit=0  Ts=0
  Product : Product
  Scope2 : Scope
  Out1 : Outport  VectorParamsAs1DForOutWhenUnconnected=off
  wires:
  [Io] -> Product/2
  Mean1/1 -> Out1/1, Scope2/1
  Product/1 -> Mean1/1
  [Vo] -> Product/1

== system DAB_variableload/BRIDGE 2/Signal Builder1 ==
  Demux : Demux  Tag=STV Demux  Outputs=1
      settings: DisplayOption=none
  FromWs : FromWorkspace  Tag=STV FromWs  VariableName=tuvar
      SigBuilderData=|
      | common.afterFinalStr = 'Extrapolate'
      | common.sampleTime = 0
      | dataSet.timeRange = [0 10]
      | dataSet.name = 'Group 1'
      | sbobj.Groups.Name = 'Group 1'
      | sbobj.Groups.Signals.Name = 'Signal 2'
      | sbobj.Groups.Signals.XData = [0 0.1 0.2 0.3 0.4 0.5 0.5 0.6 0.7 0.8 0.9 10]
      | sbobj.Groups.Signals.YData = [393 393 393 393 393 393 484 484 350 350 350 30]
  Signal 2 : Outport  Tag=STV Outport  VectorParamsAs1DForOutWhenUnconnected=off
  wires:
  FromWs/1 -> Demux/1
  Demux/1 -> Signal 2/1

== system DAB_variableload/BRIDGE 2/Signal Builder2 ==
  Demux : Demux  Tag=STV Demux  Outputs=1
      settings: DisplayOption=none
  FromWs : FromWorkspace  Tag=STV FromWs  VariableName=tuvar
      SigBuilderData=|
      | common.afterFinalStr = 'Extrapolate'
      | common.sampleTime = 0
      | dataSet.timeRange = [0 10]
      | dataSet.name = 'Group 1'
      | sbobj.Groups.Name = 'Group 1'
      | sbobj.Groups.Signals.Name = 'Signal 2'
      | sbobj.Groups.Signals.XData = [0 0.1 0.2 0.3 0.4 0.5 0.5 0.6 0.7 0.8 0.9 10]
      | sbobj.Groups.Signals.YData = [393 393 393 393 393 393 350 350 350 350 350 30]
  Signal 2 : Outport  Tag=STV Outport  VectorParamsAs1DForOutWhenUnconnected=off
  wires:
  FromWs/1 -> Demux/1
  Demux/1 -> Signal 2/1

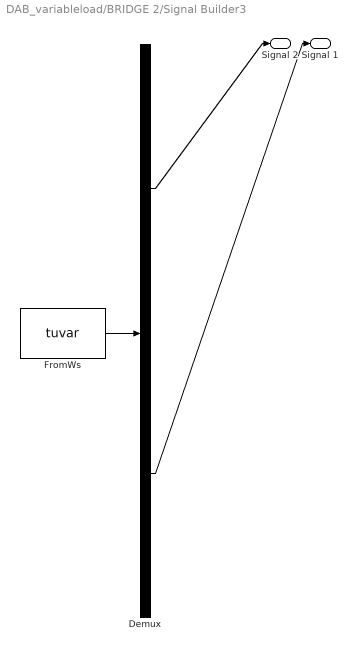
== system DAB_variableload/BRIDGE 2/Signal Builder3 ==
  Demux : Demux  Tag=STV Demux  Outputs=2
      settings: DisplayOption=none
  FromWs : FromWorkspace  Tag=STV FromWs  VariableName=tuvar
      SigBuilderData=|
      | common.afterFinalStr = 'Extrapolate'
      | common.sampleTime = 0
      | dataSet.timeRange = [0 10]
      | dataSet.name = 'Group 1'
      | sbobj.Groups.Name = 'Group 1'
      | sbobj.Groups.Signals(1).Name = 'Signal 2'
      | sbobj.Groups.Signals(1).XData = [0 0.1 0.2 0.3 0.4 0.5 0.5 0.6 0.7 0.8 0.9 10]
      | sbobj.Groups.Signals(1).YData = [31.2 31.2 31.2 31.2 31.2 31.2 15 15 15 15 15 15]
      | sbobj.Groups.Signals(2).Name = 'Signal 1'
      | sbobj.Groups.Signals(2).XData = [0 9.5 9.5 10]
      | sbobj.Groups.Signals(2).YData = [35 35 1 1]
  Signal 2 : Outport  Tag=STV Outport  VectorParamsAs1DForOutWhenUnconnected=off
  Signal 1 : Outport  Tag=STV Outport  Port=2  VectorParamsAs1DForOutWhenUnconnected=off
  wires:
  FromWs/1 -> Demux/1
  Demux/1 -> Signal 2/1
  Demux/2 -> Signal 1/1

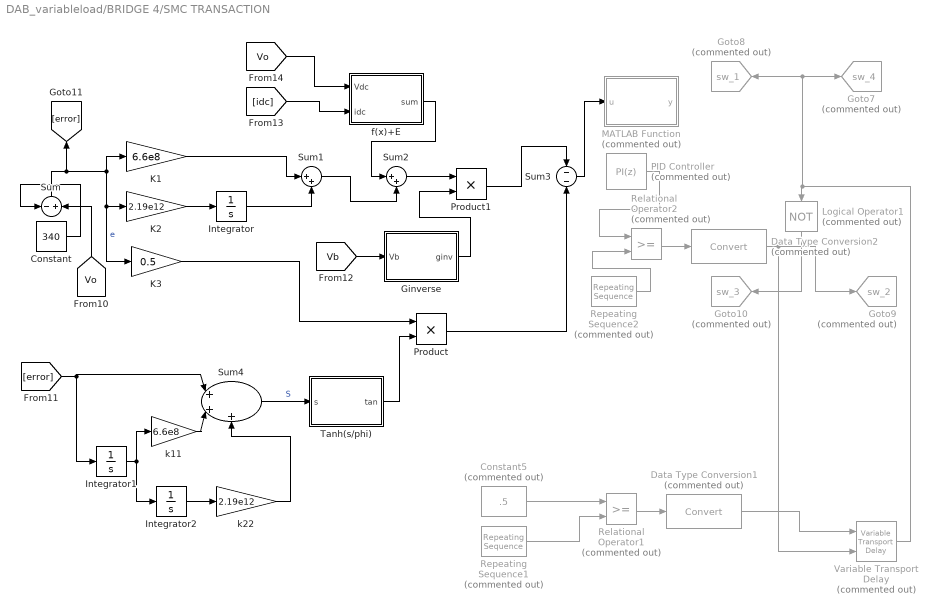
== system DAB_variableload/BRIDGE 4/SMC TRANSACTION ==
  Constant : Constant  Value=340
  Constant5 : Constant  Commented=on  Value=.5
  Data Type Conversion1 : DataTypeConversion  Commented=on  SaturateOnIntegerOverflow=off  RndMeth=Floor
  Data Type Conversion2 : DataTypeConversion  Commented=on  SaturateOnIntegerOverflow=off  RndMeth=Floor
  Ginverse : MATLAB Function  TreatAsAtomicUnit=on
  Goto10 : Goto  Commented=on  GotoTag=sw_3  TagVisibility=global
  Goto7 : Goto  Commented=on  GotoTag=sw_4  TagVisibility=global
  Goto8 : Goto  Commented=on  GotoTag=sw_1  TagVisibility=global
  Goto9 : Goto  Commented=on  GotoTag=sw_2  TagVisibility=global
  Integrator : Integrator
  Integrator1 : Integrator
  Integrator2 : Integrator
  K1 : Gain  Gain=6.6e8
  K2 : Gain  Gain=2.19e12
  K3 : Gain  Gain=0.5
  Logical Operator1 : Logic  Commented=on  Operator=NOT  AllPortsSameDT=off  OutDataTypeStr=boolean
  MATLAB Function : MATLAB Function  Commented=on  TreatAsAtomicUnit=on
  PID Controller : simulink/Continuous/PID Controller  Commented=on  Controller=PI  TimeDomain=Discrete-time  SampleTime=-1  IntegratorMethod=Forward Euler  FilterMethod=Forward Euler  Form=Parallel  UseFilter=on  ControllerParametersSource=internal  P=0.0102  I=12.817  D=0  N=100  InitialConditionSource=internal  InitialConditionForIntegrator=0  InitialConditionForFilter=0  ExternalReset=none  LimitOutput=on  UpperSaturationLimit=1  LowerSaturationLimit=-1  LinearizeAsGain=on  AntiWindupMode=none  Kb=1  TrackingMode=off  Kt=1  PParamMin=[]  PParamMax=[]  IParamMin=[]  IParamMax=[]  DParamMin=[]  DParamMax=[]  NParamMin=[]  NParamMax=[]  KbParamMin=[]  KbParamMax=[]  KtParamMin=[]  KtParamMax=[]  POutMin=[]  POutMax=[]  IOutMin=[]  IOutMax=[]  DOutMin=[]  DOutMax=[]  NOutMin=[]  NOutMax=[]  KbOutMin=[]  KbOutMax=[]  KtOutMin=[]  KtOutMax=[]  IntegratorOutMin=[]  IntegratorOutMax=[]  FilterOutMin=[]  FilterOutMax=[]  SumOutMin=[]  SumOutMax=[]  SumI1OutMin=[]  SumI1OutMax=[]  SumI2OutMin=[]  SumI2OutMax=[]  SumI3OutMin=[]  SumI3OutMax=[]  SumDOutMin=[]  SumDOutMax=[]  SaturationOutMin=[]  SaturationOutMax=[]  IntegratorContinuousStateAttributes=''  IntegratorStateMustResolveToSignalObject=off  IntegratorRTWStateStorageClass=Auto  FilterContinuousStateAttributes=''  FilterStateMustResolveToSignalObject=off  FilterRTWStateStorageClass=Auto  DifferentiatorICPrevScaledInput=0  DifferentiatorOutMin=[]  DifferentiatorOutMax=[]  FilterDiffOutCoefMin=[]  FilterDiffOutCoefMax=[]  SumDenOutMin=[]  SumDenOutMax=[]  SumNumOutMin=[]  SumNumOutMax=[]  ReciprocalOutMin=[]  ReciprocalOutMax=[]  DivideOutMin=[]  DivideOutMax=[]  TunerSelectOption=Transfer Function Based (PID Tuner App)
  Product : Product
  Product1 : Product
  Relational Operator1 : RelationalOperator  Commented=on  OutDataTypeStr=boolean  InputSameDT=off
  Relational Operator2 : RelationalOperator  Commented=on  OutDataTypeStr=boolean  InputSameDT=off
  Repeating Sequence1 : simulink/Sources/Repeating Sequence  Commented=on  rep_seq_t=[0 1/20000]  rep_seq_y=[0 1]
  Repeating Sequence2 : simulink/Sources/Repeating Sequence  Commented=on  rep_seq_t=[0 1/10000]  rep_seq_y=[0 1]
  Sum : Sum  Inputs=-+
  Sum1 : Sum  Inputs=|++
  Sum2 : Sum  Inputs=|++
  Sum3 : Sum  Inputs=--
  Sum4 : Sum  Inputs=|+++
  Tanh(s/phi) : MATLAB Function  TreatAsAtomicUnit=on
  Variable Transport Delay : VariableTransportDelay  Commented=on  VariableDelayType=Variable transport delay  MaximumDelay=0.8
  f(x)+E : MATLAB Function  TreatAsAtomicUnit=on
  k11 : Gain  Gain=6.6e8
  k22 : Gain  Gain=2.19e12
  wires:
  Data Type Conversion2/1 -> Variable Transport Delay/2, Goto9/1
  K3/1 -> Product/1
  PID Controller/1 -> Relational Operator2/1
  K2/1 -> Integrator/1
  Relational Operator1/1 -> Data Type Conversion1/1
  [idc] -> f(x)+E/2(idc)
  Integrator1/1 -> Integrator2/1, k11/1
  Product1/1 -> Sum3/1
  Tanh(s/phi)/1(tan) -> Product/2
  [Vb] -> Ginverse/1(Vb)
  Relational Operator2/1 -> Data Type Conversion2/1
  Sum1/1 -> Sum2/2
  Variable Transport Delay/1 -> Goto8/1, Goto7/1, Logical Operator1/1
  Product/1 -> Sum3/2
  Integrator/1 -> Sum1/2
  Integrator2/1 -> k22/1
  Repeating Sequence1/1 -> Relational Operator1/2
  Sum/1 -> K3/1, K2/1, K1/1, [error]  "e"
  Repeating Sequence2/1 -> Relational Operator2/2
  Sum2/1 -> Product1/1
  K1/1 -> Sum1/1
  f(x)+E/1(sum) -> Sum2/1
  k22/1 -> Sum4/3
  Constant/1 -> Sum/1
  [Vo] -> f(x)+E/1(Vdc)
  Data Type Conversion1/1 -> Variable Transport Delay/1
  [error] -> Integrator1/1, Sum4/1
  k11/1 -> Sum4/2
  Sum4/1 -> Tanh(s/phi)/1(s)  "S"
  [Vo] -> Sum/2
  Ginverse/1(ginv) -> Product1/2
  Constant5/1 -> Relational Operator1/1
  Logical Operator1/1 -> Goto10/1
  Sum3/1 -> MATLAB Function/1(u)

== system DAB_variableload/BRIDGE 4/Signal Builder1 ==
  Demux : Demux  Tag=STV Demux  Outputs=1
      settings: DisplayOption=none
  FromWs : FromWorkspace  Tag=STV FromWs  VariableName=tuvar
      SigBuilderData=|
      | common.afterFinalStr = 'Extrapolate'
      | common.sampleTime = 0
      | dataSet.timeRange = [0 10]
      | dataSet.name = 'Group 1'
      | sbobj.Groups.Name = 'Group 1'
      | sbobj.Groups.Signals.Name = 'Signal 2'
      | sbobj.Groups.Signals.XData = [0 0.1 0.2 0.3 0.4 0.5 0.5 0.6 0.7 0.8 0.9 10]
      | sbobj.Groups.Signals.YData = [393 393 393 393 393 393 484 484 350 350 350 30]
  Signal 2 : Outport  Tag=STV Outport  VectorParamsAs1DForOutWhenUnconnected=off
  wires:
  FromWs/1 -> Demux/1
  Demux/1 -> Signal 2/1

== system DAB_variableload/BRIDGE 4/Signal Builder2 ==
  Demux : Demux  Tag=STV Demux  Outputs=1
      settings: DisplayOption=none
  FromWs : FromWorkspace  Tag=STV FromWs  VariableName=tuvar
      SigBuilderData=|
      | common.afterFinalStr = 'Extrapolate'
      | common.sampleTime = 0
      | dataSet.timeRange = [0 10]
      | dataSet.name = 'Group 1'
      | sbobj.Groups.Name = 'Group 1'
      | sbobj.Groups.Signals.Name = 'Signal 2'
      | sbobj.Groups.Signals.XData = [0 0.1 0.2 0.3 0.4 0.5 0.5 0.6 0.7 0.8 0.9 10]
      | sbobj.Groups.Signals.YData = [393 393 393 393 393 393 350 350 350 350 350 30]
  Signal 2 : Outport  Tag=STV Outport  VectorParamsAs1DForOutWhenUnconnected=off
  wires:
  FromWs/1 -> Demux/1
  Demux/1 -> Signal 2/1

== system DAB_variableload/BRIDGE 4/Signal Builder3 ==
  Demux : Demux  Tag=STV Demux  Outputs=2
      settings: DisplayOption=none
  FromWs : FromWorkspace  Tag=STV FromWs  VariableName=tuvar
      SigBuilderData=|
      | common.afterFinalStr = 'Extrapolate'
      | common.sampleTime = 0
      | dataSet.timeRange = [0 10]
      | dataSet.name = 'Group 1'
      | sbobj.Groups.Name = 'Group 1'
      | sbobj.Groups.Signals(1).Name = 'Signal 2'
      | sbobj.Groups.Signals(1).XData = [0 0.1 0.2 0.3 0.4 0.5 0.5 0.6 0.7 0.8 0.9 10]
      | sbobj.Groups.Signals(1).YData = [393 393 393 393 393 393 350 350 350 350 350 350]
      | sbobj.Groups.Signals(2).Name = 'Signal 1'
      | sbobj.Groups.Signals(2).XData = [0 9.5 9.5 10]
      | sbobj.Groups.Signals(2).YData = [35 35 1 1]
  Signal 2 : Outport  Tag=STV Outport  VectorParamsAs1DForOutWhenUnconnected=off
  Signal 1 : Outport  Tag=STV Outport  Port=2  VectorParamsAs1DForOutWhenUnconnected=off
  wires:
  FromWs/1 -> Demux/1
  Demux/1 -> Signal 2/1
  Demux/2 -> Signal 1/1

== matlab function DAB_variableload/BRIDGE 2/MATLAB Function ==
  data: e input; deq output; Vin input; Vo input; Ro input
function deq = fcn(e,Vin,Vo,Ro)
fs=50000;
Ls=9.8e-6;
%Ro=31.2;
x=(4*fs*Ls)/Ro;
Co=1.8e-3;
%if t<0.5
    Voref=393;
    a2_a1=(2*log(25))/(0.04*Voref);
    y=(2*Co*a2_a1*e)/Vin;
    z=(3*Vo)/(Vin*Ro);
    f=((-(Ro^(-1)))+z+y);
    f2=sqrt(((x-1)^2)-(8*fs*Ls*f));
    deq=(1-x+f2)/2;
%(log(25))/(0.04*395)
%else 
   %Voref=350;
   %a2_a1=(2*log(25))/(0.04*Voref);
   %y=(2*Co*a2_a1*e)/Vin;
   %z=(3*Vo)/(Vin*Ro);
   %f=((-(Ro^(-1)))+z+y);
   %f2=sqrt(((x-1)^2)-(8*fs*Ls*f));
   %deq=(1-x+f2)/2;
%end

== matlab function DAB_variableload/BRIDGE 2/MATLAB Function1 ==
  data: fs input; phi output
function phi = fcn(fs)
Vdcbus=800;
n=2.15;
Lk=65.66e-6;
Vbat=393;
P=10e3;
x= (8*fs*Lk*abs(P))/(n*Vbat*Vdcbus);
y=sqrt(1-x);
phi=(pi/2)*(1-y);

== matlab function DAB_variableload/MATLAB Function ==
  data: pin input; y output; pout input
function y = fcn(pin,pout)
y=(pout/pin)*100;

== matlab function DAB_variableload/BRIDGE 4/MATLAB Function ==
  data: e input; deq output; Vin input; Vo input
function deq = fcn(e,Vin,Vo)
fs=50000;
Ls=9.8e-6;
Ro=15;
x=(4*fs*Ls)/Ro;
Co=1.8e-3;
%if t<0.5
    Voref=393;
    a2_a1=(2*log(25))/(0.04*Voref);
    y=(2*Co*a2_a1*e)/Vin;
    z=(3*Vo)/(Vin*Ro);
    f=((-(Ro^(-1)))+z+y);
    f2=sqrt(((x-1)^2)-(8*fs*Ls*f));
    deq=(1-x+f2)/2;
%(log(25))/(0.04*395)
%else 
   %Voref=350;
   %a2_a1=(2*log(25))/(0.04*Voref);
   %y=(2*Co*a2_a1*e)/Vin;
   %z=(3*Vo)/(Vin*Ro);
   %f=((-(Ro^(-1)))+z+y);
   %f2=sqrt(((x-1)^2)-(8*fs*Ls*f));
   %deq=(1-x+f2)/2;
%end

== matlab function DAB_variableload/BRIDGE 4/MATLAB Function1 ==
  data: fs input; phi output
function phi = fcn(fs)
Vdcbus=800;
n=2.15;
Lk=65.66e-6;
Vbat=393;
P=10e3;
x= (8*fs*Lk*abs(P))/(n*Vbat*Vdcbus);
y=sqrt(1-x);
phi=(pi/2)*(1-y);

== matlab function DAB_variableload/BRIDGE 4/SMC TRANSACTION/Ginverse ==
  data: Vb input; ginv output
function ginv = fcn(Vb)
n=4.6;
Rs=1;
Ls=31e-6;
fs=10000;
Cdc=200e-6;
ws=2*pi*fs;
z=sqrt((Rs^2)+((ws*Ls)^2));
denom=Cdc*(pi^2)*z;
g=(8*n*Vb)/denom;
ginv=g^(-1);

== matlab function DAB_variableload/BRIDGE 4/SMC TRANSACTION/MATLAB Function ==
  data: u input; y output
function y = fcn(u)

y = -asin(u);

== matlab function DAB_variableload/BRIDGE 4/SMC TRANSACTION/Tanh(s//phi) ==
  data: s input; tan output
function tan = fcn(s)
mew=1.2e2;
tan= tanh(s/mew);

== matlab function DAB_variableload/BRIDGE 4/SMC TRANSACTION/f(x)+E ==
  data: Vdc input; sum output; idc input
function sum = fcn(Vdc,idc)
fs=10000;
ws=2*pi*fs;
Ls=31e-6;
Rs=1;
Cdc=200e-6;
phi=atan(ws*Ls/Rs);
cphi=cos(phi);
z=sqrt((Rs^2)+((ws*Ls)^2));
denom=Cdc*(pi^2)*z;
f=-(8*cphi*Vdc)/denom;
E=-(idc/Cdc);
sum=f+E;
